simulink model "lab1_model3"  (R2012b)
settings: Solver=ode45  StartTime=0.0  StopTime=100.0  RelTol=1e-3
settings Model: Creator=student-at  LastModifiedBy=student-at

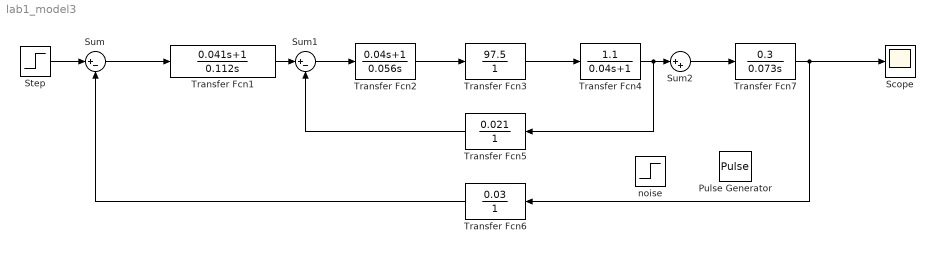
== system lab1_model3 ==
  Pulse Generator : DiscretePulseGenerator  PulseType=Time based  Amplitude=-10  Period=10
  Scope : Scope
  Step : Step  SampleTime=0
  Sum : Sum  Inputs=|+-
  Sum1 : Sum  Inputs=|+-
  Sum2 : Sum  Inputs=|++
  Transfer Fcn1 : TransferFcn  Numerator=[0.041, 1]  Denominator=[0.112 0]
  Transfer Fcn2 : TransferFcn  Numerator=[0.04, 1]  Denominator=[0.056 0]
  Transfer Fcn3 : TransferFcn  Numerator=[97.5]  Denominator=[0 1]
  Transfer Fcn4 : TransferFcn  Numerator=[1.1]  Denominator=[0.04 1]
  Transfer Fcn5 : TransferFcn  Numerator=[0.021]  Denominator=[0 1]
  Transfer Fcn6 : TransferFcn  Numerator=[0.03]  Denominator=[0 1]
  Transfer Fcn7 : TransferFcn  Numerator=[0.3]  Denominator=[0.073 0]
  noise : Step  Time=25  After=-20  SampleTime=0
  wires:
  Sum/1 -> Transfer Fcn1/1
  Transfer Fcn1/1 -> Sum1/1
  Transfer Fcn2/1 -> Transfer Fcn3/1
  Sum1/1 -> Transfer Fcn2/1
  Transfer Fcn3/1 -> Transfer Fcn4/1
  Transfer Fcn4/1 -> Transfer Fcn5/1, Sum2/1
  Transfer Fcn5/1 -> Sum1/2
  Transfer Fcn6/1 -> Sum/2
  Sum2/1 -> Transfer Fcn7/1
  Transfer Fcn7/1 -> Transfer Fcn6/1, Scope/1
  Step/1 -> Sum/1
